simulink model "BLDC_SixStep_Speed_Current_Loop_Control"  (R2022b)
settings: Solver=FixedStepDiscrete  StartTime=0.0  StopTime=1  FixedStep=1e-6  RelTol=1e-3
model workspace (MAT data in the model file):
  Ctrol_Mode = 3
  Current_Control_Mode = 2
  Current_PID_Upper_Limit = 1
  PWM_Period = 0.0001
  Speed_I = 2
  Speed_P = 6
  Speed_PID_Upper_Limit = 19
  Ts_time = 1e-06
  current_I = 0.2
  current_P = 3
libraries: simulink x18, slpidlib x3, eePwmGenerator x3, spsPermanentMagnetSynchronousMachineLib x1, spsDCVoltageSourceLib x1, spsTwoLevelConverterLib x1, spspowerguiLib x1
settings Model: Creator=31904  LastModifiedBy=31904

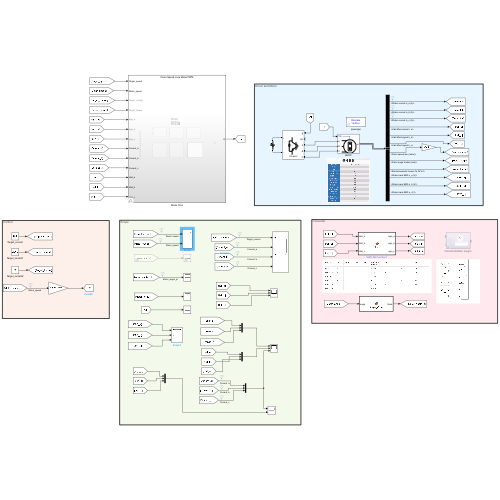
[thumbnail: Simulink's stored preview of the top-level diagram]
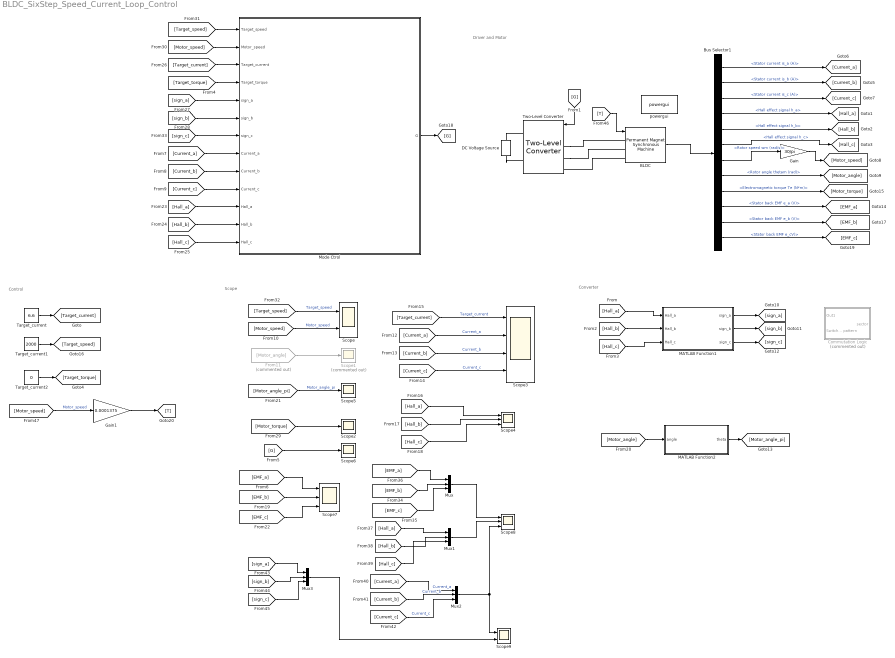
== system BLDC_SixStep_Speed_Current_Loop_Control ==
  note: Converter
  note: Control
  note: Scope
  note: Driver and Motor
  BLDC : spsPermanentMagnetSynchronousMachineLib/Permanent Magnet Synchronous Machine  NbPhases=3  FluxDistribution=Trapezoidal  RotorType=Round  MechanicalLoad=Torque Tm  PresetModel=No  ShowDetailedParameters=on  MeasurementBus=off  Resistance=0.2  Inductance=0.0004  dqInductances=[8.5e-3,8.5e-3]  La=0.0004  MachineConstant=Torque Constant (N.m / A_peak)  Flux=0.01575  VoltageCst=6.5973  TorqueCst=0.063  Flat=120  Mechanical=[2.1e-05 0 2]  PolePairs=4  InitialConditions=[0,0, 0,0]  InitialConditions5ph=[0 0 0 0 0 0]  RefAngle=Aligned with phase A axis (original Park)  IterativeDiscreteModel=Trapezoidal non iterative  TsBlock=-1  TsPowergui=0
  Bus Selector1 : BusSelector  OutputSignals=Stator current is_a (A),Stator current is_b (A),Stator current is_c (A),Hall effect signal h_a,Hall effect signal h_b,Hall effect signal h_c,Rotor speed wm (rad/s),Rotor angle thetam (rad),Electromagnetic torque Te (N*m),Stator back EMF e_a (V),Stator back EMF e_b (V),Stator back EMF e_cV)
  Commutation Logic : Subsystem  Commented=on
  DC Voltage Source : spsDCVoltageSourceLib/DC Voltage Source  Amplitude=24  Measurements=None
  From11 : From  Commented=on  GotoTag=Motor_angle
  Gain : Gain  Gain=30/pi
  Gain1 : Gain  Gain=0.0001375
  MATLAB Function1 : MATLAB Function  TreatAsAtomicUnit=on
  MATLAB Function2 : MATLAB Function  TreatAsAtomicUnit=on
  Mode Ctrol : Subsystem  Variant=on
  Mux{,1..3} (4 alike) : Mux  Inputs=3
  Scope : Scope  NumInputPorts=2
  Scope1 : Scope  Commented=on
  Scope2 : Scope
  Scope3 : Scope  NumInputPorts=4
  Scope4 : Scope  NumInputPorts=3
  Scope5 : Scope
  Scope6 : Scope
  Scope7 : Scope  NumInputPorts=3
  Scope8 : Scope  NumInputPorts=3
  Scope9 : Scope  NumInputPorts=2
  Target_current : Constant  Value=6.6
  Target_current1 : Constant  Value=2000
  Target_current2 : Constant  Value=0
  Two-Level Converter : spsTwoLevelConverterLib/Two-Level Converter  ModelType=Switching devices  Ron=0.0001  Rs=1e6  Cs=inf  Vforward=[0,0]  Ron_Diode=1e-3  Rs_Diode=1e6  Cs_Diode=inf  Vf_Diode=1e-3  Rs_CurrentSource=inf  Ron_ACsource=1e-3
  powergui : spspowerguiLib/powergui  Priority=1  SimulationMode=Discrete  SampleTime=0.000001  frequency=60  Iterations=50  frequencyindice=0  Pbase=100e6  ErrMax=1e-4  UnitsV=kV  UnitsW=MW  buscounter=0  FunctionMessages=off  echomessages=off  EnableUseOfTLC=off  CurrentSourceSwitches=off  DisableSnubberDevices=off  DisableRonSwitches=off  DisableVfSwitches=off  DisplayEquations=off  AutomaticDiscreteSolvers=off  SolverType=Tustin/Backward Euler (TBE)  Interpol=off  ExternalGateDelay=off  methode=off  Ts=100  x0status=blocks  SPID=on  SwTol=0  HookPort=off  NonlinearTolerance=1e-4  nMaxIteration=100  ContinueOnMaxIteration=off  RestoreLinks=warning  ResistiveCurrentMeasurement=off  Frange=[0:2:500]  Ylog=off  Xlog=on  ShowGrid=off  save=off  variable=ZData  structure=0  ZoomFFT=off  StartTime=0.0  cycles=1  DisplayStyle=1  fundamental=60  FreqAxis=off  MaxFrequency=1000  frequencyindicesteady=1  RmsSteady=1  display=off
  wires:
  [T] -> BLDC/1
  [G] -> Two-Level Converter/1
  Bus Selector1/3 -> [Current_c]  "<Stator current is_c (A)>"
  Bus Selector1/8 -> [Motor_angle]  "<Rotor angle thetam (rad)>"
  Bus Selector1/1 -> [Current_a]  "<Stator current is_a (A)>"
  Bus Selector1/6 -> [Hall_c]  "<Hall effect signal h_c>"
  Bus Selector1/4 -> [Hall_a]  "<Hall effect signal h_a>"
  Bus Selector1/2 -> [Current_b]  "<Stator current is_b (A)>"
  Bus Selector1/7 -> Gain/1  "<Rotor speed wm (rad/s)>"
  Bus Selector1/5 -> [Hall_b]  "<Hall effect signal h_b>"
  BLDC/1 -> Bus Selector1/1
  [Hall_a] -> MATLAB Function1/1(Hall_a)
  [Hall_b] -> MATLAB Function1/2(Hall_b)
  [Hall_c] -> MATLAB Function1/3(Hall_c)
  MATLAB Function1/1(sign_a) -> [sign_a]
  MATLAB Function1/2(sign_b) -> [sign_b]
  MATLAB Function1/3(sign_c) -> [sign_c]
  [Motor_speed] -> Scope/2  "Motor_speed"
  [Current_a] -> Scope3/2  "Current_a"
  [Current_b] -> Scope3/3  "Current_b"
  [Current_c] -> Scope3/4  "Current_c"
  [Target_current] -> Scope3/1  "Target_current"
  [Hall_a] -> Scope4/1
  [Hall_b] -> Scope4/2
  [Hall_c] -> Scope4/3
  From11/1 -> Scope1/1
  [Motor_angle] -> MATLAB Function2/1(angle)
  [Motor_angle_pi] -> Scope5/1  "Motor_angle_pi"
  MATLAB Function2/1(theta) -> [Motor_angle_pi]
  Bus Selector1/9 -> [Motor_torque]  "<Electromagnetic torque Te (N*m)>"
  [Motor_torque] -> Scope2/1
  Target_current1/1 -> [Target_speed]
  [Target_speed] -> Scope/1  "Target_speed"
  Mode Ctrol/1(G) -> [G]
  [sign_a] -> Mode Ctrol/5(sign_a)
  [sign_b] -> Mode Ctrol/6(sign_b)
  [sign_c] -> Mode Ctrol/7(sign_c)
  [Target_current] -> Mode Ctrol/3(Target_current)
  [Target_speed] -> Mode Ctrol/1(Target_speed)
  [Motor_speed] -> Mode Ctrol/2(Motor_speed)
  [Target_torque] -> Mode Ctrol/4(Target_torque)
  Target_current2/1 -> [Target_torque]
  [Current_a] -> Mode Ctrol/8(Current_a)
  [Current_b] -> Mode Ctrol/9(Current_b)
  [Current_c] -> Mode Ctrol/10(Current_c)
  Gain/1 -> [Motor_speed]
  [G] -> Scope6/1
  Bus Selector1/10 -> [EMF_a]  "<Stator back EMF e_a (V)>"
  Bus Selector1/11 -> [EMF_b]  "<Stator back EMF e_b (V)>"
  Bus Selector1/12 -> [EMF_c]  "<Stator back EMF e_cV)>"
  [EMF_a] -> Scope7/1
  [EMF_b] -> Scope7/2
  [EMF_c] -> Scope7/3
  [Hall_a] -> Mode Ctrol/11(Hall_a)
  [Hall_b] -> Mode Ctrol/12(Hall_b)
  [Hall_c] -> Mode Ctrol/13(Hall_c)
  [EMF_a] -> Mux/1
  [EMF_b] -> Mux/2
  [EMF_c] -> Mux/3
  [Hall_a] -> Mux1/1
  [Hall_b] -> Mux1/2
  [Hall_c] -> Mux1/3
  Mux1/1 -> Scope8/2
  [Current_a] -> Mux2/1  "Current_a"
  [Current_b] -> Mux2/2  "Current_b"
  [Current_c] -> Mux2/3  "Current_c"
  Mux/1 -> Scope8/1
  Mux2/1 -> Scope8/3, Scope9/1
  Target_current/1 -> [Target_current]
  [sign_a] -> Mux3/1
  [sign_b] -> Mux3/2
  [sign_c] -> Mux3/3
  Mux3/1 -> Scope9/2
  [Motor_speed] -> Gain1/1  "Motor_speed"
  Gain1/1 -> [T]
  connections:
  Two-Level Converter/LConn2 -- BLDC/LConn2
  BLDC/LConn3 -- Two-Level Converter/LConn3
  Two-Level Converter/LConn1 -- BLDC/LConn1
  DC Voltage Source/LConn1 -- Two-Level Converter/RConn2
  DC Voltage Source/RConn1 -- Two-Level Converter/RConn1

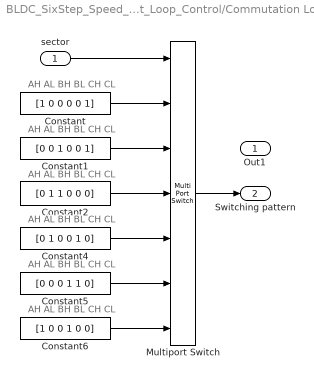
== system BLDC_SixStep_Speed_Current_Loop_Control/Commutation Logic ==
  note: AH AL BH BL CH CL
  note: AH AL BH BL CH CL
  note: AH AL BH BL CH CL
  note: AH AL BH BL CH CL
  note: AH AL BH BL CH CL
  note: AH AL BH BL CH CL
  sector : Inport
  Constant : Constant  Value=[1 0 0 0 0 1]
  Constant1 : Constant  Value=[0 0 1 0 0 1]
  Constant2 : Constant  Value=[0 1 1 0 0 0]
  Constant4 : Constant  Value=[0 1 0 0 1 0]
  Constant5 : Constant  Value=[0 0 0 1 1 0]
  Constant6 : Constant  Value=[1 0 0 1 0 0]
  Multiport Switch : MultiPortSwitch  Inputs=6  SaturateOnIntegerOverflow=off  InputSameDT=off
  Out1 : Outport
  "  Switching pattern" : Outport  Port=2  VectorParamsAs1DForOutWhenUnconnected=off
  wires:
  Constant4/1 -> Multiport Switch/5
  Constant5/1 -> Multiport Switch/6
  Constant6/1 -> Multiport Switch/7
  sector/1 -> Multiport Switch/1
  Constant2/1 -> Multiport Switch/4
  Multiport Switch/1 -> "  Switching pattern"/1
  Constant1/1 -> Multiport Switch/3
  Constant/1 -> Multiport Switch/2

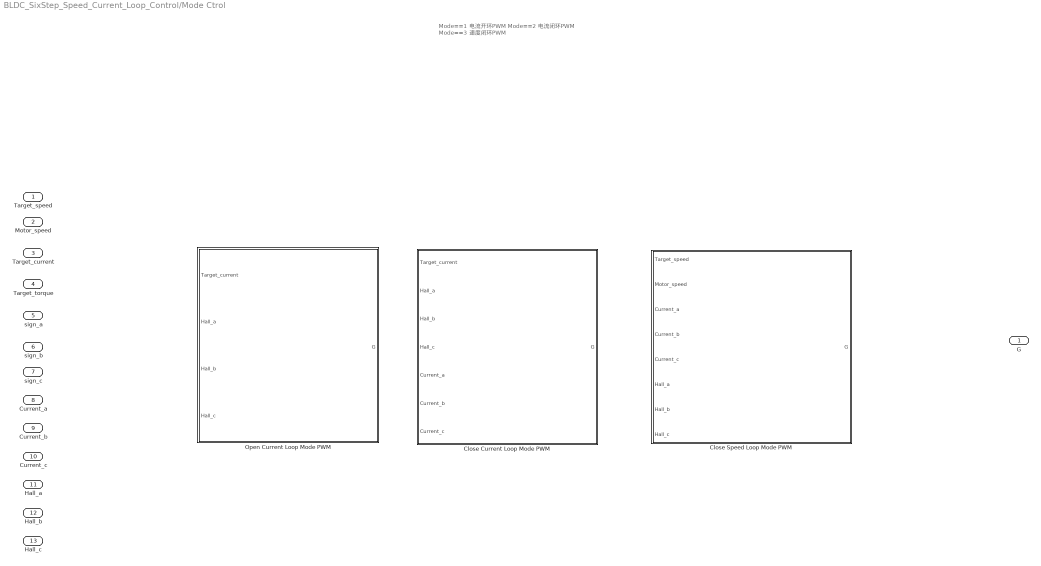
== system BLDC_SixStep_Speed_Current_Loop_Control/Mode Ctrol ==
  note: Mode==1 电流开环PWM
      | Mode==2 电流闭环PWM
      | Mode==3 速度闭环PWM
  Target_speed : Inport
  Motor_speed : Inport  Port=2
  Target_current : Inport  Port=3
  Target_torque : Inport  Port=4
  sign_a : Inport  Port=5
  sign_b : Inport  Port=6
  sign_c : Inport  Port=7
  Current_a : Inport  Port=8
  Current_b : Inport  Port=9
  Current_c : Inport  Port=10
  Hall_a : Inport  Port=11
  Hall_b : Inport  Port=12
  Hall_c : Inport  Port=13
  Close Current Loop Mode PWM : Subsystem  TreatAsAtomicUnit=on  VariantControl=Ctrol_Mode==2
  Close Speed Loop Mode PWM : Subsystem  TreatAsAtomicUnit=on  VariantControl=Ctrol_Mode==3
  Open Current Loop Mode PWM : Subsystem  TreatAsAtomicUnit=on  VariantControl=Ctrol_Mode==1
  G : Outport

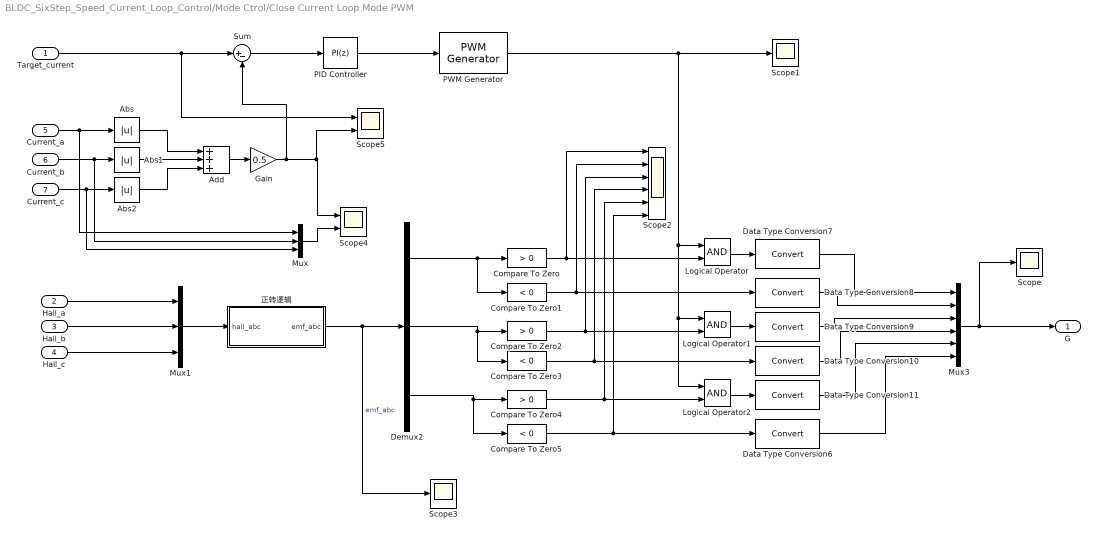
== system BLDC_SixStep_Speed_Current_Loop_Control/Mode Ctrol/Close Current Loop Mode PWM ==
  Target_current : Inport
  Hall_a : Inport  Port=2
  Hall_b : Inport  Port=3
  Hall_c : Inport  Port=4
  Current_a : Inport  Port=5
  Current_b : Inport  Port=6
  Current_c : Inport  Port=7
  Abs : Abs  SaturateOnIntegerOverflow=off
  Abs1 : Abs  SaturateOnIntegerOverflow=off
  Abs2 : Abs  SaturateOnIntegerOverflow=off
  Add : Sum  Inputs=+++
  Compare To Zero : simulink/Logic and Bit Operations/Compare To Zero  relop=>  OutDataTypeStr=boolean  ZeroCross=off
  Compare To Zero1 : simulink/Logic and Bit Operations/Compare To Zero  relop=<  OutDataTypeStr=boolean  ZeroCross=off
  Compare To Zero2 : simulink/Logic and Bit Operations/Compare To Zero  relop=>  OutDataTypeStr=boolean  ZeroCross=off
  Compare To Zero3 : simulink/Logic and Bit Operations/Compare To Zero  relop=<  OutDataTypeStr=boolean  ZeroCross=off
  Compare To Zero4 : simulink/Logic and Bit Operations/Compare To Zero  relop=>  OutDataTypeStr=boolean  ZeroCross=off
  Compare To Zero5 : simulink/Logic and Bit Operations/Compare To Zero  relop=<  OutDataTypeStr=boolean  ZeroCross=off
  Data Type Conversion{6..11} (6 alike) : DataTypeConversion  SaturateOnIntegerOverflow=off  RndMeth=Floor
  Demux2 : Demux  Outputs=3
  Gain : Gain  Gain=0.5
  Logical Operator : Logic  AllPortsSameDT=off  OutDataTypeStr=boolean
  Logical Operator1 : Logic  AllPortsSameDT=off  OutDataTypeStr=boolean
  Logical Operator2 : Logic  AllPortsSameDT=off  OutDataTypeStr=boolean
  Mux : Mux  Inputs=3
  Mux1 : Mux  Inputs=3
  Mux3 : Mux  Inputs=6
  PID Controller : slpidlib/PID Controller  Controller=PI  Form=Parallel  TimeDomain=Discrete-time  UseExternalTs=off  SampleTime=-1  IntegratorMethod=Forward Euler  FilterMethod=Forward Euler  ControllerParametersSource=internal  P=current_P  I=current_I  UseKiTs=off  D=0  N=100  UseFilter=on  TunerSelectOption=Transfer Function Based (PID Tuner App)  InitialConditionSource=internal  InitialConditionForIntegrator=0  InitialConditionForFilter=0  DifferentiatorICPrevScaledInput=0  ExternalReset=none  TrackingMode=off  Kt=1  LimitOutput=on  SatLimitsSource=internal  UpperSaturationLimit=1  LowerSaturationLimit=0  LinearizeAsGain=on  AntiWindupMode=none  Kb=1  LimitIntegrator=off  UpperIntegratorSaturationLimit=inf  LowerIntegratorSaturationLimit=-inf  POutMin=[]  POutMax=[]  IOutMin=[]  IOutMax=[]  DOutMin=[]  DOutMax=[]  NOutMin=[]  NOutMax=[]  SumOutMin=[]  SumOutMax=[]  SaturationOutMin=[]  SaturationOutMax=[]  PParamMin=[]  PParamMax=[]  IParamMin=[]  IParamMax=[]  DParamMin=[]  DParamMax=[]  NParamMin=[]  NParamMax=[]  KbParamMin=[]  KbParamMax=[]  KtParamMin=[]  KtParamMax=[]  KbOutMin=[]  KbOutMax=[]  KtOutMin=[]  KtOutMax=[]  IntegratorOutMin=[]  IntegratorOutMax=[]  FilterOutMin=[]  FilterOutMax=[]  SumI1OutMin=[]  SumI1OutMax=[]  SumI2OutMin=[]  SumI2OutMax=[]  SumI3OutMin=[]  SumI3OutMax=[]  SumI4OutMin=[]  SumI4OutMax=[]  SumDOutMin=[]  SumDOutMax=[]  DifferentiatorOutMin=[]  DifferentiatorOutMax=[]  FilterDiffOutCoefMin=[]  FilterDiffOutCoefMax=[]  ReciprocalOutMin=[]  ReciprocalOutMax=[]  SumDenOutMin=[]  SumDenOutMax=[]  SumNumOutMin=[]  SumNumOutMax=[]  DivideOutMin=[]  DivideOutMax=[]  UdiffTsProdOutMin=[]  UdiffTsProdOutMax=[]  NTsProdOutMin=[]  NTsProdOutMax=[]  UintegralTsProdOutMin=[]  UintegralTsProdOutMax=[]  UngainTsProdOutMin=[]  UngainTsProdOutMax=[]  ClampingZeroOutDataTypeStr=Inherit: Inherit via back propagation  ClampingZeroOutMin=[]  ClampingZeroOutMax=[]  FilterDenConstantOutDataTypeStr=Inherit: Inherit via back propagation  FilterDenConstantOutMin=[]  FilterDenConstantOutMax=[]  PCopyOutDataTypeStr=Inherit: Inherit via back propagation  PCopyOutMin=[]  PCopyOutMax=[]  NCopyOutDataTypeStr=Inherit: Inherit via back propagation  NCopyOutMin=[]  NCopyOutMax=[]  IntegratorContinuousStateAttributes=''  IntegratorStateMustResolveToSignalObject=off  IntegratorRTWStateStorageClass=Auto  FilterContinuousStateAttributes=''  FilterStateMustResolveToSignalObject=off  FilterRTWStateStorageClass=Auto  ParallelPVariant=InternalParameters  IdealPVariant=Disabled  IVariant=InternalParameters  DVariant=Disabled  IntegratorVariant=Discrete  SatVariant=Enabled  AWVariant=Passthrough  PCopyVariant=Disabled  TRVariant=Disabled  FdbkBlocksVariant=Forward  IdealPFdbkVariant=Disabled  SatFdbkVariant=Disabled  DerivativeFilterVariant=Disabled  NVariant=Disabled  NCopyVariant=Disabled_SignalSpec  FilterICVariant=Disabled  IntegratorICVariant=InternalICs  ExternalResetVariant=Disabled  TRSumVariant=Passthrough  SumFdbkVariant=Disabled  SumVariant=Sum_PI  TsampFilterVariant=InternalTs  TsampNgainVariant=Passthrough  TsampIntegralVariant=Passthrough  ExternalSaturationOutDataTypeStr=Inherit: Same as second input
  PWM Generator : eePwmGenerator/PWM Generator  CarrCount=Up  Tper=PWM_Period  Tdelay=0  Ts=Ts_time
  Scope : Scope
  Scope1 : Scope
  Scope2 : Scope  NumInputPorts=6
  Scope3 : Scope
  Scope4 : Scope  NumInputPorts=2
  Scope5 : Scope  NumInputPorts=2
  Sum : Sum  Inputs=|+-
  正转逻辑 : Subsystem
  G : Outport
  wires:
  PWM Generator/1 -> Logical Operator/1, Logical Operator1/1, Logical Operator2/1, Scope1/1
  Compare To Zero3/1 -> Data Type Conversion10/1, Scope2/4
  Demux2/2 -> Compare To Zero2/1, Compare To Zero3/1
  Mux3/1 -> Scope/1, G/1
  Demux2/3 -> Compare To Zero5/1, Compare To Zero4/1
  Logical Operator1/1 -> Data Type Conversion9/1
  Compare To Zero4/1 -> Logical Operator2/2, Scope2/5
  Compare To Zero2/1 -> Logical Operator1/2, Scope2/3
  Logical Operator2/1 -> Data Type Conversion11/1
  Demux2/1 -> Compare To Zero1/1, Compare To Zero/1
  Compare To Zero/1 -> Logical Operator/2, Scope2/1
  Logical Operator/1 -> Data Type Conversion7/1
  Compare To Zero1/1 -> Data Type Conversion8/1, Scope2/2
  Compare To Zero5/1 -> Data Type Conversion6/1, Scope2/6
  正转逻辑/1(emf_abc) -> Scope3/1, Demux2/1  "emf_abc"
  Hall_a/1 -> Mux1/1
  Hall_b/1 -> Mux1/2
  Hall_c/1 -> Mux1/3
  Mux1/1 -> 正转逻辑/1(hall_abc)
  Data Type Conversion7/1 -> Mux3/1
  Data Type Conversion8/1 -> Mux3/2
  Data Type Conversion9/1 -> Mux3/3
  Data Type Conversion10/1 -> Mux3/4
  Data Type Conversion11/1 -> Mux3/5
  Data Type Conversion6/1 -> Mux3/6
  Current_a/1 -> Abs/1, Mux/1
  Abs/1 -> Add/1
  Current_b/1 -> Mux/2, Abs1/1
  Abs1/1 -> Add/2
  Current_c/1 -> Mux/3, Abs2/1
  Abs2/1 -> Add/3
  Add/1 -> Gain/1
  PID Controller/1 -> PWM Generator/1
  Gain/1 -> Sum/2, Scope5/2, Scope4/1
  Mux/1 -> Scope4/2
  Sum/1 -> PID Controller/1
  Target_current/1 -> Scope5/1, Sum/1

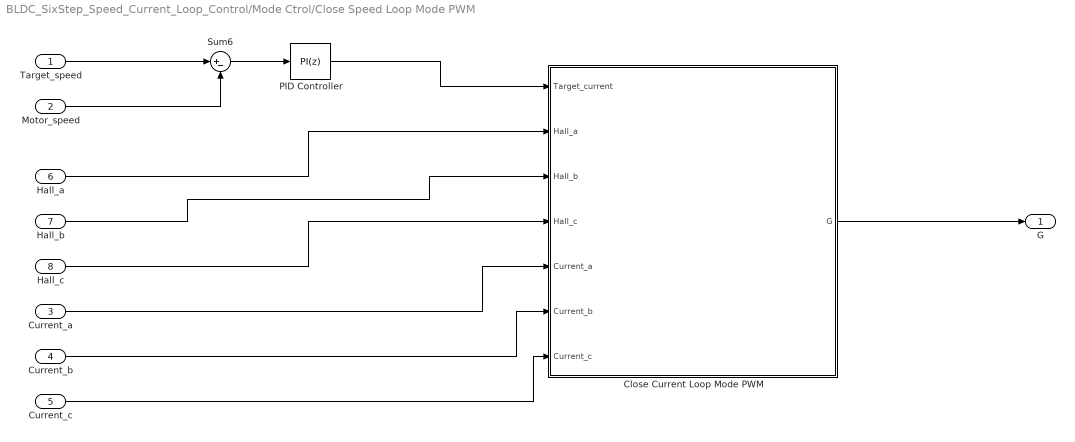
== system BLDC_SixStep_Speed_Current_Loop_Control/Mode Ctrol/Close Speed Loop Mode PWM ==
  Target_speed : Inport
  Motor_speed : Inport  Port=2
  Current_a : Inport  Port=3
  Current_b : Inport  Port=4
  Current_c : Inport  Port=5
  Hall_a : Inport  Port=6
  Hall_b : Inport  Port=7
  Hall_c : Inport  Port=8
  Close Current Loop Mode PWM : Subsystem  TreatAsAtomicUnit=on  VariantControl=Ctrol_Mode==5
  PID Controller : slpidlib/PID Controller  Controller=PI  Form=Parallel  TimeDomain=Discrete-time  UseExternalTs=off  SampleTime=-1  IntegratorMethod=Forward Euler  FilterMethod=Forward Euler  ControllerParametersSource=internal  P=Speed_P  I=Speed_I  UseKiTs=off  D=0  N=100  UseFilter=on  TunerSelectOption=Transfer Function Based (PID Tuner App)  InitialConditionSource=internal  InitialConditionForIntegrator=0  InitialConditionForFilter=0  DifferentiatorICPrevScaledInput=0  ExternalReset=none  TrackingMode=off  Kt=1  LimitOutput=on  SatLimitsSource=internal  UpperSaturationLimit=Speed_PID_Upper_Limit  LowerSaturationLimit=0  LinearizeAsGain=off  AntiWindupMode=clamping  Kb=1  LimitIntegrator=off  UpperIntegratorSaturationLimit=inf  LowerIntegratorSaturationLimit=-inf  POutMin=[]  POutMax=[]  IOutMin=[]  IOutMax=[]  DOutMin=[]  DOutMax=[]  NOutMin=[]  NOutMax=[]  SumOutMin=[]  SumOutMax=[]  SaturationOutMin=[]  SaturationOutMax=[]  PParamMin=[]  PParamMax=[]  IParamMin=[]  IParamMax=[]  DParamMin=[]  DParamMax=[]  NParamMin=[]  NParamMax=[]  KbParamMin=[]  KbParamMax=[]  KtParamMin=[]  KtParamMax=[]  KbOutMin=[]  KbOutMax=[]  KtOutMin=[]  KtOutMax=[]  IntegratorOutMin=[]  IntegratorOutMax=[]  FilterOutMin=[]  FilterOutMax=[]  SumI1OutMin=[]  SumI1OutMax=[]  SumI2OutMin=[]  SumI2OutMax=[]  SumI3OutMin=[]  SumI3OutMax=[]  SumI4OutMin=[]  SumI4OutMax=[]  SumDOutMin=[]  SumDOutMax=[]  DifferentiatorOutMin=[]  DifferentiatorOutMax=[]  FilterDiffOutCoefMin=[]  FilterDiffOutCoefMax=[]  ReciprocalOutMin=[]  ReciprocalOutMax=[]  SumDenOutMin=[]  SumDenOutMax=[]  SumNumOutMin=[]  SumNumOutMax=[]  DivideOutMin=[]  DivideOutMax=[]  UdiffTsProdOutMin=[]  UdiffTsProdOutMax=[]  NTsProdOutMin=[]  NTsProdOutMax=[]  UintegralTsProdOutMin=[]  UintegralTsProdOutMax=[]  UngainTsProdOutMin=[]  UngainTsProdOutMax=[]  ClampingZeroOutDataTypeStr=Inherit: Inherit via back propagation  ClampingZeroOutMin=[]  ClampingZeroOutMax=[]  FilterDenConstantOutDataTypeStr=Inherit: Inherit via back propagation  FilterDenConstantOutMin=[]  FilterDenConstantOutMax=[]  PCopyOutDataTypeStr=Inherit: Inherit via back propagation  PCopyOutMin=[]  PCopyOutMax=[]  NCopyOutDataTypeStr=Inherit: Inherit via back propagation  NCopyOutMin=[]  NCopyOutMax=[]  IntegratorContinuousStateAttributes=''  IntegratorStateMustResolveToSignalObject=off  IntegratorRTWStateStorageClass=Auto  FilterContinuousStateAttributes=''  FilterStateMustResolveToSignalObject=off  FilterRTWStateStorageClass=Auto  ParallelPVariant=InternalParameters  IdealPVariant=Disabled  IVariant=InternalParameters  DVariant=Disabled  IntegratorVariant=Discrete  SatVariant=Enabled  AWVariant=DiscClampingParallel  PCopyVariant=Disabled  TRVariant=Disabled  FdbkBlocksVariant=Forward  IdealPFdbkVariant=Disabled  SatFdbkVariant=Disabled  DerivativeFilterVariant=Disabled  NVariant=Disabled  NCopyVariant=Disabled_SignalSpec  FilterICVariant=Disabled  IntegratorICVariant=InternalICs  ExternalResetVariant=Disabled  TRSumVariant=Passthrough  SumFdbkVariant=Disabled  SumVariant=Sum_PI  TsampFilterVariant=InternalTs  TsampNgainVariant=Passthrough  TsampIntegralVariant=Passthrough  ExternalSaturationOutDataTypeStr=Inherit: Same as second input
  Sum6 : Sum  Inputs=|+-
  G : Outport
  wires:
  Current_a/1 -> Close Current Loop Mode PWM/5(Current_a)
  Current_c/1 -> Close Current Loop Mode PWM/7(Current_c)
  Current_b/1 -> Close Current Loop Mode PWM/6(Current_b)
  Close Current Loop Mode PWM/1(G) -> G/1
  PID Controller/1 -> Close Current Loop Mode PWM/1(Target_current)
  Motor_speed/1 -> Sum6/2
  Target_speed/1 -> Sum6/1
  Sum6/1 -> PID Controller/1
  Hall_a/1 -> Close Current Loop Mode PWM/2(Hall_a)
  Hall_b/1 -> Close Current Loop Mode PWM/3(Hall_b)
  Hall_c/1 -> Close Current Loop Mode PWM/4(Hall_c)

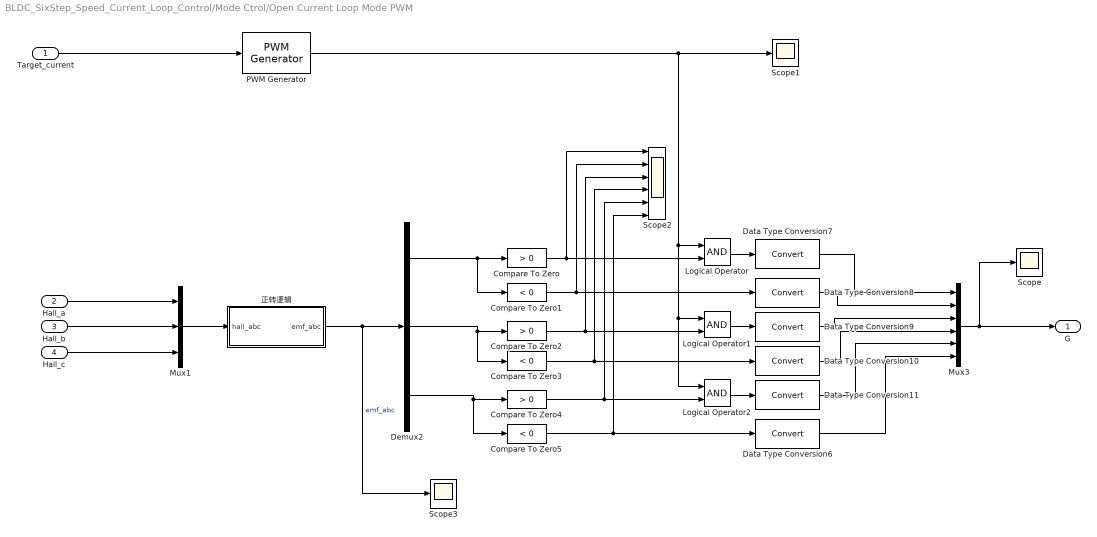
== system BLDC_SixStep_Speed_Current_Loop_Control/Mode Ctrol/Open Current Loop Mode PWM ==
  Target_current : Inport
  Hall_a : Inport  Port=2
  Hall_b : Inport  Port=3
  Hall_c : Inport  Port=4
  Compare To Zero : simulink/Logic and Bit Operations/Compare To Zero  relop=>  OutDataTypeStr=boolean  ZeroCross=off
  Compare To Zero1 : simulink/Logic and Bit Operations/Compare To Zero  relop=<  OutDataTypeStr=boolean  ZeroCross=off
  Compare To Zero2 : simulink/Logic and Bit Operations/Compare To Zero  relop=>  OutDataTypeStr=boolean  ZeroCross=off
  Compare To Zero3 : simulink/Logic and Bit Operations/Compare To Zero  relop=<  OutDataTypeStr=boolean  ZeroCross=off
  Compare To Zero4 : simulink/Logic and Bit Operations/Compare To Zero  relop=>  OutDataTypeStr=boolean  ZeroCross=off
  Compare To Zero5 : simulink/Logic and Bit Operations/Compare To Zero  relop=<  OutDataTypeStr=boolean  ZeroCross=off
  Data Type Conversion{6..11} (6 alike) : DataTypeConversion  SaturateOnIntegerOverflow=off  RndMeth=Floor
  Demux2 : Demux  Outputs=3
  Logical Operator : Logic  AllPortsSameDT=off  OutDataTypeStr=boolean
  Logical Operator1 : Logic  AllPortsSameDT=off  OutDataTypeStr=boolean
  Logical Operator2 : Logic  AllPortsSameDT=off  OutDataTypeStr=boolean
  Mux1 : Mux  Inputs=3
  Mux3 : Mux  Inputs=6
  PWM Generator : eePwmGenerator/PWM Generator  CarrCount=Up  Tper=PWM_Period  Tdelay=0  Ts=Ts_time
  Scope : Scope
  Scope1 : Scope
  Scope2 : Scope  NumInputPorts=6
  Scope3 : Scope
  正转逻辑 : Subsystem
  G : Outport
  wires:
  Data Type Conversion6/1 -> Mux3/6
  Data Type Conversion11/1 -> Mux3/5
  Data Type Conversion10/1 -> Mux3/4
  Data Type Conversion9/1 -> Mux3/3
  Data Type Conversion8/1 -> Mux3/2
  Data Type Conversion7/1 -> Mux3/1
  Mux1/1 -> 正转逻辑/1(hall_abc)
  Hall_c/1 -> Mux1/3
  Hall_b/1 -> Mux1/2
  Hall_a/1 -> Mux1/1
  正转逻辑/1(emf_abc) -> Demux2/1, Scope3/1  "emf_abc"
  Compare To Zero5/1 -> Scope2/6, Data Type Conversion6/1
  Compare To Zero1/1 -> Scope2/2, Data Type Conversion8/1
  Logical Operator/1 -> Data Type Conversion7/1
  Compare To Zero/1 -> Scope2/1, Logical Operator/2
  Demux2/1 -> Compare To Zero/1, Compare To Zero1/1
  Logical Operator2/1 -> Data Type Conversion11/1
  Compare To Zero2/1 -> Scope2/3, Logical Operator1/2
  Compare To Zero4/1 -> Scope2/5, Logical Operator2/2
  Logical Operator1/1 -> Data Type Conversion9/1
  Demux2/3 -> Compare To Zero4/1, Compare To Zero5/1
  Mux3/1 -> G/1, Scope/1
  Demux2/2 -> Compare To Zero3/1, Compare To Zero2/1
  Compare To Zero3/1 -> Scope2/4, Data Type Conversion10/1
  Target_current/1 -> PWM Generator/1
  PWM Generator/1 -> Scope1/1, Logical Operator2/1, Logical Operator1/1, Logical Operator/1

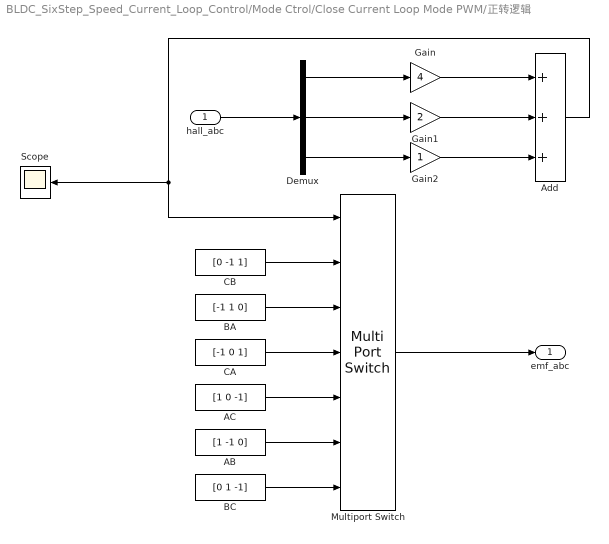
== system BLDC_SixStep_Speed_Current_Loop_Control/Mode Ctrol/Close Current Loop Mode PWM/正转逻辑 ==
  hall_abc : Inport
  AB : Constant  Value=[1 -1 0]
  AC : Constant  Value=[1 0 -1]
  Add : Sum  Inputs=+++
  BA : Constant  Value=[-1 1 0]
  BC : Constant  Value=[0 1 -1]
  CA : Constant  Value=[-1 0 1]
  CB : Constant  Value=[0 -1 1]
  Demux : Demux  Outputs=3
  Gain : Gain  Gain=4
  Gain1 : Gain  Gain=2
  Gain2 : Gain
  Multiport Switch : MultiPortSwitch  Inputs=6  SaturateOnIntegerOverflow=off  InputSameDT=off
  Scope : Scope
  emf_abc : Outport
  wires:
  BA/1 -> Multiport Switch/3
  CB/1 -> Multiport Switch/2
  CA/1 -> Multiport Switch/4
  AB/1 -> Multiport Switch/6
  BC/1 -> Multiport Switch/7
  Multiport Switch/1 -> emf_abc/1
  Add/1 -> Scope/1, Multiport Switch/1
  AC/1 -> Multiport Switch/5
  Gain/1 -> Add/1
  Gain1/1 -> Add/2
  Gain2/1 -> Add/3
  Demux/2 -> Gain1/1
  Demux/1 -> Gain/1
  Demux/3 -> Gain2/1
  hall_abc/1 -> Demux/1

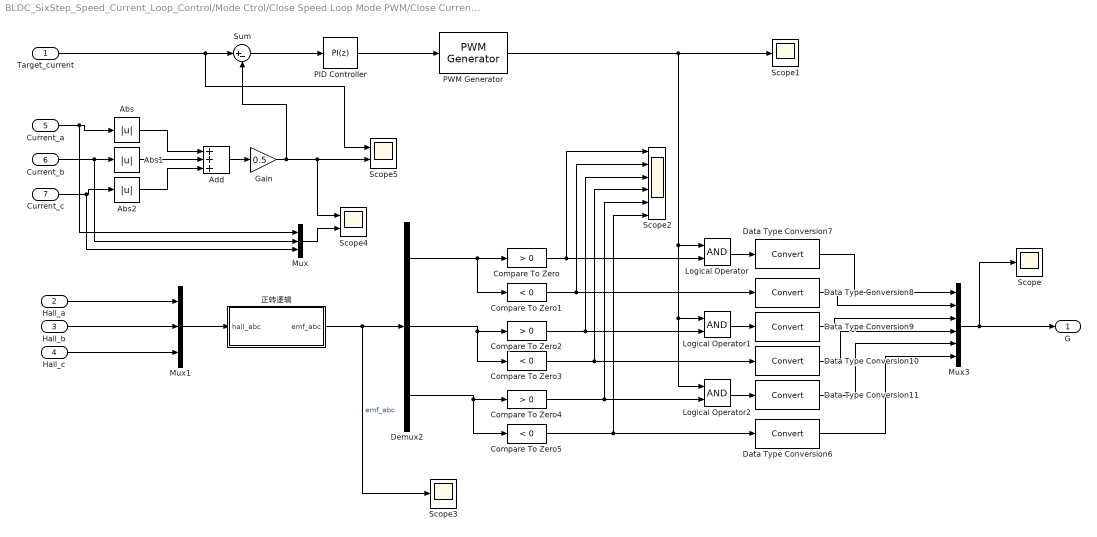
== system BLDC_SixStep_Speed_Current_Loop_Control/Mode Ctrol/Close Speed Loop Mode PWM/Close Current Loop Mode PWM ==
  Target_current : Inport
  Hall_a : Inport  Port=2
  Hall_b : Inport  Port=3
  Hall_c : Inport  Port=4
  Current_a : Inport  Port=5
  Current_b : Inport  Port=6
  Current_c : Inport  Port=7
  Abs : Abs  SaturateOnIntegerOverflow=off
  Abs1 : Abs  SaturateOnIntegerOverflow=off
  Abs2 : Abs  SaturateOnIntegerOverflow=off
  Add : Sum  Inputs=+++
  Compare To Zero : simulink/Logic and Bit Operations/Compare To Zero  relop=>  OutDataTypeStr=boolean  ZeroCross=off
  Compare To Zero1 : simulink/Logic and Bit Operations/Compare To Zero  relop=<  OutDataTypeStr=boolean  ZeroCross=off
  Compare To Zero2 : simulink/Logic and Bit Operations/Compare To Zero  relop=>  OutDataTypeStr=boolean  ZeroCross=off
  Compare To Zero3 : simulink/Logic and Bit Operations/Compare To Zero  relop=<  OutDataTypeStr=boolean  ZeroCross=off
  Compare To Zero4 : simulink/Logic and Bit Operations/Compare To Zero  relop=>  OutDataTypeStr=boolean  ZeroCross=off
  Compare To Zero5 : simulink/Logic and Bit Operations/Compare To Zero  relop=<  OutDataTypeStr=boolean  ZeroCross=off
  Data Type Conversion{6..11} (6 alike) : DataTypeConversion  SaturateOnIntegerOverflow=off  RndMeth=Floor
  Demux2 : Demux  Outputs=3
  Gain : Gain  Gain=0.5
  Logical Operator : Logic  AllPortsSameDT=off  OutDataTypeStr=boolean
  Logical Operator1 : Logic  AllPortsSameDT=off  OutDataTypeStr=boolean
  Logical Operator2 : Logic  AllPortsSameDT=off  OutDataTypeStr=boolean
  Mux : Mux  Inputs=3
  Mux1 : Mux  Inputs=3
  Mux3 : Mux  Inputs=6
  PID Controller : slpidlib/PID Controller  Controller=PI  Form=Parallel  TimeDomain=Discrete-time  UseExternalTs=off  SampleTime=-1  IntegratorMethod=Forward Euler  FilterMethod=Forward Euler  ControllerParametersSource=internal  P=current_P  I=current_I  UseKiTs=off  D=0  N=100  UseFilter=on  TunerSelectOption=Transfer Function Based (PID Tuner App)  InitialConditionSource=internal  InitialConditionForIntegrator=0  InitialConditionForFilter=0  DifferentiatorICPrevScaledInput=0  ExternalReset=none  TrackingMode=off  Kt=1  LimitOutput=on  SatLimitsSource=internal  UpperSaturationLimit=1  LowerSaturationLimit=0  LinearizeAsGain=on  AntiWindupMode=none  Kb=1  LimitIntegrator=off  UpperIntegratorSaturationLimit=inf  LowerIntegratorSaturationLimit=-inf  POutMin=[]  POutMax=[]  IOutMin=[]  IOutMax=[]  DOutMin=[]  DOutMax=[]  NOutMin=[]  NOutMax=[]  SumOutMin=[]  SumOutMax=[]  SaturationOutMin=[]  SaturationOutMax=[]  PParamMin=[]  PParamMax=[]  IParamMin=[]  IParamMax=[]  DParamMin=[]  DParamMax=[]  NParamMin=[]  NParamMax=[]  KbParamMin=[]  KbParamMax=[]  KtParamMin=[]  KtParamMax=[]  KbOutMin=[]  KbOutMax=[]  KtOutMin=[]  KtOutMax=[]  IntegratorOutMin=[]  IntegratorOutMax=[]  FilterOutMin=[]  FilterOutMax=[]  SumI1OutMin=[]  SumI1OutMax=[]  SumI2OutMin=[]  SumI2OutMax=[]  SumI3OutMin=[]  SumI3OutMax=[]  SumI4OutMin=[]  SumI4OutMax=[]  SumDOutMin=[]  SumDOutMax=[]  DifferentiatorOutMin=[]  DifferentiatorOutMax=[]  FilterDiffOutCoefMin=[]  FilterDiffOutCoefMax=[]  ReciprocalOutMin=[]  ReciprocalOutMax=[]  SumDenOutMin=[]  SumDenOutMax=[]  SumNumOutMin=[]  SumNumOutMax=[]  DivideOutMin=[]  DivideOutMax=[]  UdiffTsProdOutMin=[]  UdiffTsProdOutMax=[]  NTsProdOutMin=[]  NTsProdOutMax=[]  UintegralTsProdOutMin=[]  UintegralTsProdOutMax=[]  UngainTsProdOutMin=[]  UngainTsProdOutMax=[]  ClampingZeroOutDataTypeStr=Inherit: Inherit via back propagation  ClampingZeroOutMin=[]  ClampingZeroOutMax=[]  FilterDenConstantOutDataTypeStr=Inherit: Inherit via back propagation  FilterDenConstantOutMin=[]  FilterDenConstantOutMax=[]  PCopyOutDataTypeStr=Inherit: Inherit via back propagation  PCopyOutMin=[]  PCopyOutMax=[]  NCopyOutDataTypeStr=Inherit: Inherit via back propagation  NCopyOutMin=[]  NCopyOutMax=[]  IntegratorContinuousStateAttributes=''  IntegratorStateMustResolveToSignalObject=off  IntegratorRTWStateStorageClass=Auto  FilterContinuousStateAttributes=''  FilterStateMustResolveToSignalObject=off  FilterRTWStateStorageClass=Auto  ParallelPVariant=InternalParameters  IdealPVariant=Disabled  IVariant=InternalParameters  DVariant=Disabled  IntegratorVariant=Discrete  SatVariant=Enabled  AWVariant=Passthrough  PCopyVariant=Disabled  TRVariant=Disabled  FdbkBlocksVariant=Forward  IdealPFdbkVariant=Disabled  SatFdbkVariant=Disabled  DerivativeFilterVariant=Disabled  NVariant=Disabled  NCopyVariant=Disabled_SignalSpec  FilterICVariant=Disabled  IntegratorICVariant=InternalICs  ExternalResetVariant=Disabled  TRSumVariant=Passthrough  SumFdbkVariant=Disabled  SumVariant=Sum_PI  TsampFilterVariant=InternalTs  TsampNgainVariant=Passthrough  TsampIntegralVariant=Passthrough  ExternalSaturationOutDataTypeStr=Inherit: Same as second input
  PWM Generator : eePwmGenerator/PWM Generator  CarrCount=Up  Tper=PWM_Period  Tdelay=0  Ts=Ts_time
  Scope : Scope
  Scope1 : Scope
  Scope2 : Scope  NumInputPorts=6
  Scope3 : Scope
  Scope4 : Scope  NumInputPorts=2
  Scope5 : Scope  NumInputPorts=2
  Sum : Sum  Inputs=|+-
  正转逻辑 : Subsystem
  G : Outport
  wires:
  PWM Generator/1 -> Logical Operator/1, Logical Operator1/1, Logical Operator2/1, Scope1/1
  Compare To Zero3/1 -> Data Type Conversion10/1, Scope2/4
  Demux2/2 -> Compare To Zero2/1, Compare To Zero3/1
  Mux3/1 -> Scope/1, G/1
  Demux2/3 -> Compare To Zero5/1, Compare To Zero4/1
  Logical Operator1/1 -> Data Type Conversion9/1
  Compare To Zero4/1 -> Logical Operator2/2, Scope2/5
  Compare To Zero2/1 -> Logical Operator1/2, Scope2/3
  Logical Operator2/1 -> Data Type Conversion11/1
  Demux2/1 -> Compare To Zero1/1, Compare To Zero/1
  Compare To Zero/1 -> Logical Operator/2, Scope2/1
  Logical Operator/1 -> Data Type Conversion7/1
  Compare To Zero1/1 -> Data Type Conversion8/1, Scope2/2
  Compare To Zero5/1 -> Data Type Conversion6/1, Scope2/6
  正转逻辑/1(emf_abc) -> Scope3/1, Demux2/1  "emf_abc"
  Hall_a/1 -> Mux1/1
  Hall_b/1 -> Mux1/2
  Hall_c/1 -> Mux1/3
  Mux1/1 -> 正转逻辑/1(hall_abc)
  Data Type Conversion7/1 -> Mux3/1
  Data Type Conversion8/1 -> Mux3/2
  Data Type Conversion9/1 -> Mux3/3
  Data Type Conversion10/1 -> Mux3/4
  Data Type Conversion11/1 -> Mux3/5
  Data Type Conversion6/1 -> Mux3/6
  Current_a/1 -> Mux/1, Abs/1
  Abs/1 -> Add/1
  Current_b/1 -> Mux/2, Abs1/1
  Abs1/1 -> Add/2
  Current_c/1 -> Mux/3, Abs2/1
  Abs2/1 -> Add/3
  Add/1 -> Gain/1
  PID Controller/1 -> PWM Generator/1
  Gain/1 -> Sum/2, Scope5/2, Scope4/1
  Mux/1 -> Scope4/2
  Sum/1 -> PID Controller/1
  Target_current/1 -> Scope5/1, Sum/1

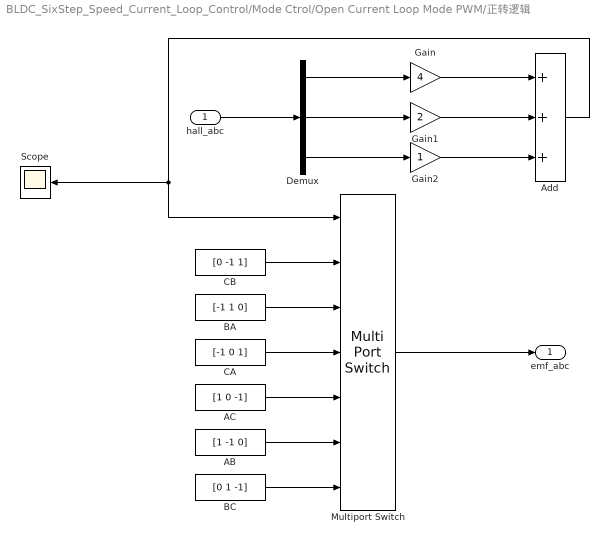
== system BLDC_SixStep_Speed_Current_Loop_Control/Mode Ctrol/Open Current Loop Mode PWM/正转逻辑 ==
  hall_abc : Inport
  AB : Constant  Value=[1 -1 0]
  AC : Constant  Value=[1 0 -1]
  Add : Sum  Inputs=+++
  BA : Constant  Value=[-1 1 0]
  BC : Constant  Value=[0 1 -1]
  CA : Constant  Value=[-1 0 1]
  CB : Constant  Value=[0 -1 1]
  Demux : Demux  Outputs=3
  Gain : Gain  Gain=4
  Gain1 : Gain  Gain=2
  Gain2 : Gain
  Multiport Switch : MultiPortSwitch  Inputs=6  SaturateOnIntegerOverflow=off  InputSameDT=off
  Scope : Scope
  emf_abc : Outport
  wires:
  hall_abc/1 -> Demux/1
  Demux/3 -> Gain2/1
  Demux/1 -> Gain/1
  Demux/2 -> Gain1/1
  Gain2/1 -> Add/3
  Gain1/1 -> Add/2
  Gain/1 -> Add/1
  AC/1 -> Multiport Switch/5
  Add/1 -> Multiport Switch/1, Scope/1
  Multiport Switch/1 -> emf_abc/1
  BC/1 -> Multiport Switch/7
  AB/1 -> Multiport Switch/6
  CA/1 -> Multiport Switch/4
  CB/1 -> Multiport Switch/2
  BA/1 -> Multiport Switch/3

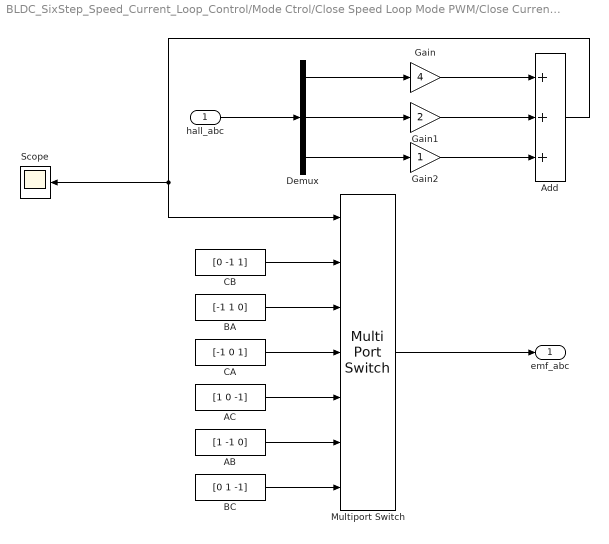
== system BLDC_SixStep_Speed_Current_Loop_Control/Mode Ctrol/Close Speed Loop Mode PWM/Close Current Loop Mode PWM/正转逻辑 ==
  hall_abc : Inport
  AB : Constant  Value=[1 -1 0]
  AC : Constant  Value=[1 0 -1]
  Add : Sum  Inputs=+++
  BA : Constant  Value=[-1 1 0]
  BC : Constant  Value=[0 1 -1]
  CA : Constant  Value=[-1 0 1]
  CB : Constant  Value=[0 -1 1]
  Demux : Demux  Outputs=3
  Gain : Gain  Gain=4
  Gain1 : Gain  Gain=2
  Gain2 : Gain
  Multiport Switch : MultiPortSwitch  Inputs=6  SaturateOnIntegerOverflow=off  InputSameDT=off
  Scope : Scope
  emf_abc : Outport
  wires:
  BA/1 -> Multiport Switch/3
  CB/1 -> Multiport Switch/2
  CA/1 -> Multiport Switch/4
  AB/1 -> Multiport Switch/6
  BC/1 -> Multiport Switch/7
  Multiport Switch/1 -> emf_abc/1
  Add/1 -> Scope/1, Multiport Switch/1
  AC/1 -> Multiport Switch/5
  Gain/1 -> Add/1
  Gain1/1 -> Add/2
  Gain2/1 -> Add/3
  Demux/2 -> Gain1/1
  Demux/1 -> Gain/1
  Demux/3 -> Gain2/1
  hall_abc/1 -> Demux/1

== matlab function BLDC_SixStep_Speed_Current_Loop_Control/MATLAB Function2 ==
  data: angle input; theta output
function theta = Angle_Conv(angle)

n=mod(angle,pi);

theta = n;

== matlab function BLDC_SixStep_Speed_Current_Loop_Control/MATLAB Function1 ==
  data: Hall_a input; sign_a output; Hall_b input; Hall_c input; sign_b output; sign_c output
function [sign_a,sign_b,sign_c] = fcn(Hall_a, Hall_b, Hall_c)

if Hall_a==1&&Hall_b==0&&Hall_c==1

sign_a=1;
sign_b=0;
sign_c=-1;

elseif Hall_a==1&&Hall_b==0&&Hall_c==0

sign_a=0;
sign_b=1;
sign_c=-1;


elseif Hall_a==1&&Hall_b==1&&Hall_c==0

sign_a=-1;
sign_b=1;
sign_c=0;


elseif Hall_a==0&&Hall_b==1&&Hall_c==0

sign_a=-1;
sign_b=0;
sign_c=1;


elseif Hall_a==0&&Hall_b==1&&Hall_c==1

sign_a=0;
sign_b=-1;
sign_c=1;

else

sign_a=1;
sign_b=-1;
sign_c=0;


end
